simulink model "test_mpu6000_02"  (Simulink 8.8)
settings: Solver=FixedStepDiscrete  StartTime=0.0  StopTime=10.0  FixedStep=0.01  RelTol=1e-3  EnableMultiTasking=on
InitFcn:
  | px4_ap1_mdl_callback('check_model');
undefined symbols (not defined in the file or in its folder): s
libraries: px4_ap1_mpu_6000_lib x1, px4_ap1_px4setup_lib x1
settings Model: Creator=Privat  LastModifiedBy=Privat
settings OptimizationCC: ExpressionDepthLimit=2147483647  InitFltsAndDblsToZero=on  LifeSpan=1
settings DebuggingCC: SolverPrmCheckMsg=warning  InheritedTsInSrcMsg=none  StrictBusMsg=Warning
settings RTWCC: SystemTargetFile=px4_ap1.tlc  GenCodeOnly=on  GenerateMakefile=off
settings CodeAppCC: IgnoreCustomStorageClasses=off  CustomSymbolStrType=$N$R$M  InternalIdentifier=Classic
settings STFCustomTargetCC: ModelReferenceCompliant=off  IncludeMdlTerminateFcn=off  CombineOutputUpdateFcns=on  ERTCustomFileBanners=on  SupportContinuousTime=off  SupportNonInlinedSFcns=off  RemoveResetFunc=on  MATLABClassNameForMDSCustomization=Simulink.SoftwareTarget.ERTCustomization  CPPClassGenCompliant=on  GRTInterface=off  SystemTargetFile=px4_ap1.tlc
settings ERTTargetCC: MultiwordLength=2048  ModelReferenceCompliant=off  ParMdlRefBuildCompliant=off  CompOptLevelCompliant=off  ConcurrentExecutionCompliant=off  IncludeMdlTerminateFcn=off  ERTFirstTimeCompliant=off  ModelStepFunctionPrototypeControlCompliant=off  UseToolchainInfoCompliant=off  ERTSrcFileBannerTemplate=px4_ap1_code_template.cgt  ERTHdrFileBannerTemplate=px4_ap1_code_template.cgt  ERTDataSrcFileTemplate=px4_ap1_code_template.cgt  ERTDataHdrFileTemplate=px4_ap1_code_template.cgt  ERTCustomFileTemplate=px4_ap1_main.tlc  ConvertIfToSwitch=off  SuppressUnreachableDefaultCases=off

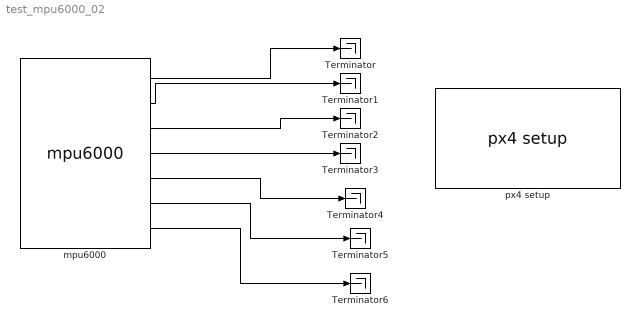
== system test_mpu6000_02 ==
  Terminator{,1..6} (7 alike) : Terminator
  mpu6000 : px4_ap1_mpu_6000_lib/mpu6000  Description=Setup for PX4 native software  accelRange=+/- 16g  gyroRange=2000°/s  filter=5Hz  accXcorr=1  accYcorr=1  accZcorr=1  accXoff=0  accYoff=0  accZoff=0
  px4 setup : px4_ap1_px4setup_lib/px4 setup  SampleTimeValue=0.01  cbBuild=on  cbUpload=off  cbPort=COM0  cpuLoad=off  debugmode=on
  wires:
  mpu6000/1 -> Terminator/1
  mpu6000/2 -> Terminator1/1
  mpu6000/3 -> Terminator2/1
  mpu6000/4 -> Terminator3/1
  mpu6000/5 -> Terminator4/1
  mpu6000/6 -> Terminator5/1
  mpu6000/7 -> Terminator6/1
